simulink model "modelo_lti_d_residual"  (R2022b)
settings: Solver=VariableStepAuto  StartTime=0.0  StopTime=10.0  RelTol=1e-3
values from neighbouring files (symbols this model uses):
  b_eq = b_eq_max    (= 2.40277777778e-05)    [analisis_estabilidad.m]    (also in parametros.m = 2.19444444444e-05; parametros_sim.m = 2.19444444444e-05)
  C_ts = 0.818    [analisis_estabilidad.m]    (also in parametros.m; parametros_sim.m)
  J_eq = J_eq_max    (= 4.58263888889e-05)    [analisis_estabilidad.m]    (also in parametros.m = 1.97847222222e-05; parametros_sim.m = 1.97847222222e-05)
  L_q = 5.8    [analisis_estabilidad.m]    (also in parametros.m = 0.0058; parametros_sim.m; polosyceros.m = L_q^3)
  lambda_m = 0.016    [analisis_estabilidad.m]    (also in parametros.m; parametros_sim.m)
  P_p = 3    [analisis_estabilidad.m]    (also in parametros.m; parametros_sim.m)
  r = 120    [analisis_estabilidad.m]    (also in parametros.m; parametros_sim.m)
  R_s = R_s_max    (= 1.39791)    [analisis_estabilidad.m]    (also in frec_nat_y_amort.m = R_s_ref * (1 + alpha_Cu * (T - T_s_ref)); parametros.m = 1.02)
  R_ts_amb = 146.7    [analisis_estabilidad.m]    (also in parametros.m; parametros_sim.m)
settings Model: Creator=martinarobyculasso  LastModifiedBy=martinarobyculasso

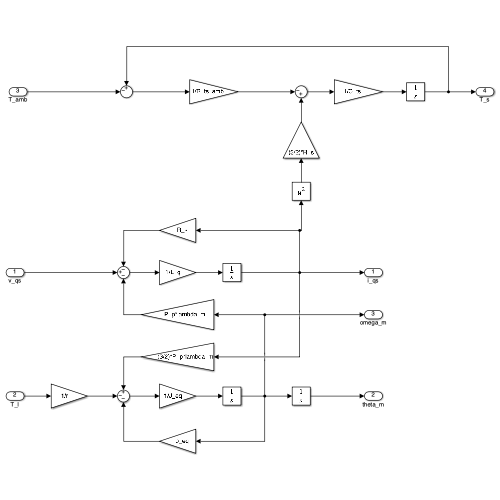
[thumbnail: Simulink's stored preview of the top-level diagram]
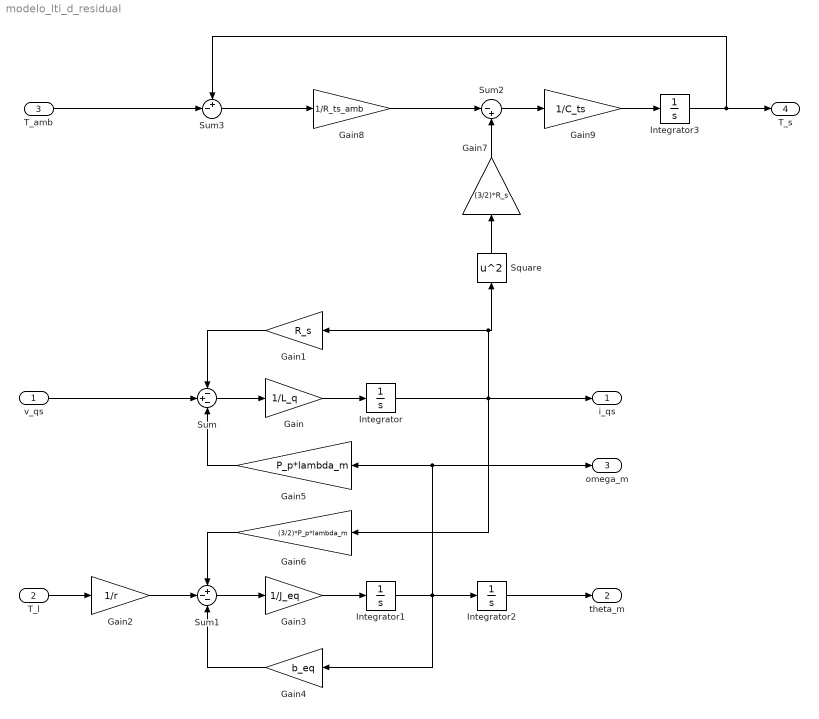
== system modelo_lti_d_residual ==
  v_qs : Inport
  T_l : Inport  Port=2
  T_amb : Inport  Port=3
  Gain : Gain  Gain=1/L_q
  Gain1 : Gain  Gain=R_s
  Gain2 : Gain  Gain=1/r
  Gain3 : Gain  Gain=1/J_eq
  Gain4 : Gain  Gain=b_eq
  Gain5 : Gain  Gain=P_p*lambda_m
  Gain6 : Gain  Gain=(3/2)*P_p*lambda_m
  Gain7 : Gain  Gain=(3/2)*R_s
  Gain8 : Gain  Gain=1/R_ts_amb
  Gain9 : Gain  Gain=1/C_ts
  Integrator{,1..3} (4 alike) : Integrator
  Square : Math  Operator=square
  Sum : Sum  Inputs=-+-
  Sum1 : Sum  Inputs=+--
  Sum2 : Sum  Inputs=|-+
  Sum3 : Sum  Inputs=+-|
  i_qs : Outport
  theta_m : Outport  Port=2
  omega_m : Outport  Port=3
  T_s : Outport  Port=4
  wires:
  v_qs/1 -> Sum/2
  Sum/1 -> Gain/1
  Gain/1 -> Integrator/1
  Gain1/1 -> Sum/1
  Integrator/1 -> Gain6/1, i_qs/1, Gain1/1, Square/1
  T_l/1 -> Gain2/1
  Gain2/1 -> Sum1/2
  Sum1/1 -> Gain3/1
  Gain3/1 -> Integrator1/1
  Integrator1/1 -> Gain4/1, omega_m/1, Gain5/1, Integrator2/1
  Integrator2/1 -> theta_m/1
  Gain4/1 -> Sum1/3
  Gain5/1 -> Sum/3
  Gain6/1 -> Sum1/1
  Square/1 -> Gain7/1
  Gain7/1 -> Sum2/2
  T_amb/1 -> Sum3/2
  Sum3/1 -> Gain8/1
  Gain8/1 -> Sum2/1
  Sum2/1 -> Gain9/1
  Integrator3/1 -> Sum3/1, T_s/1
  Gain9/1 -> Integrator3/1
